simulink model "CASMain"  (R2023b)
settings: Solver=FixedStepAuto  StartTime=0.0  StopTime=10.0  FixedStep=0.01  RelTol=1e-3
values from neighbouring files (symbols this model uses):
  aircraft_mass = 5    [ACConfig.m]
  center_of_gravity = [0 0 0]    [ACConfig.m]
  center_of_pressure = [0 0 0]    [ACConfig.m]
  max_aileron_deflection = 30    [ACConfig.m]
  max_elevator_deflection = 30    [ACConfig.m]
  max_rudder_deflection = 30    [ACConfig.m]
  max_throttle = 100.0    (= 100)    [ACConfig.m]
  plane_latitude = 45    [ACConfig.m]
  plane_longitude = 45    [ACConfig.m]
undefined symbols (not defined in the file or in its folder): magnitude
libraries: aerolibasang x2, sim3dcameralib x2, shared6dof x1, aerolibatmos2 x1, dspmathops x1, sim3dphyssensorlib x1, sim3dlib x1, uavsim3dlib x1
settings Model: Creator=burak  LastModifiedBy=burak

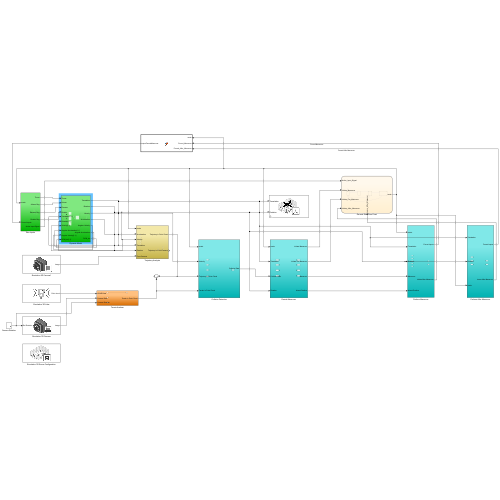
[thumbnail: Simulink's stored preview of the top-level diagram]
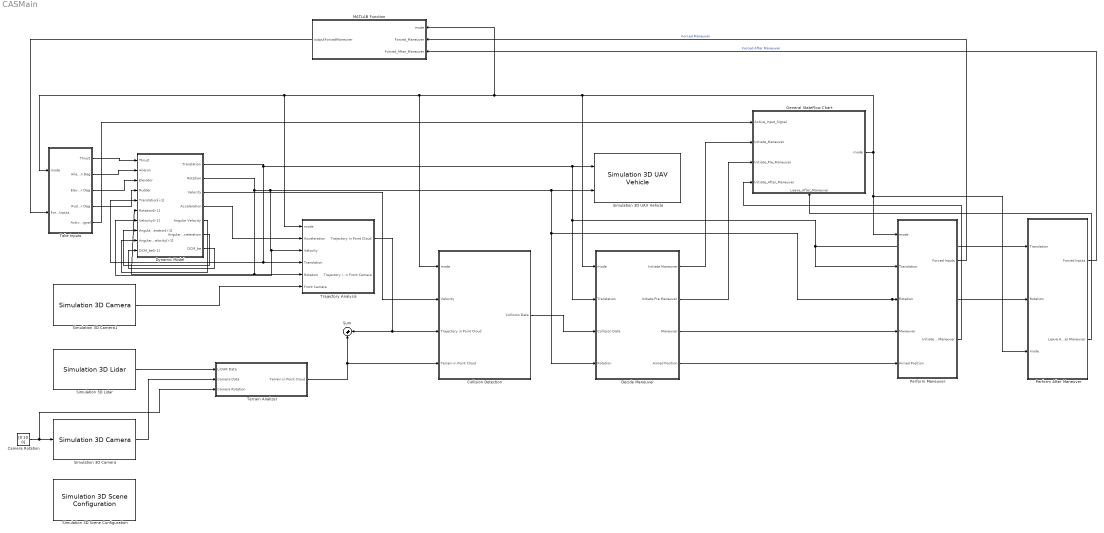
== system CASMain ==
  Camera Rotation : Constant  Value=[0 10 0]  VectorParams1D=off
  Collision Detection : Subsystem
  Decide Maneuver : Subsystem
  Dynamic Model : Subsystem
  General StateFlow Chart : Stateflow chart  TreatAsAtomicUnit=on
      settings: PortSchema="{\"entries\":[{\"content\":{\"sides\":[{\"content\":{\"connectorIds\":[\"In2\",\"In3\",\"In4\",\"In5\"]},\"type\":\"ConnectorPlacement.EquallySpacedRectSide\",\"uuid\":\"7a30dc9d-b2d0-4cd8-a09a-60d22ea8c87b\"},{\"content\":{\"connectorIds\":[\"Out1\"],\"side\":\"RIGHT\"},\"type\":\"ConnectorPlacement.EquallySpacedRectSide\",\"uuid\":\"c8b32d95-5109-4e90-83c3-dc864e15907c\"},{\"content\":{\"side\":\"TOP\"},\"type\":\"ConnectorPlacement.EquallySpacedRectSide\",\"uuid\":\"64dca0b5-bb3e-47b4-89ff-52a03a0aa1bb\"},{\"content\":{\"connectorIds\":[\"In1\"],\"side\":\"BOTTOM\"},\"type\":\"ConnectorPlacement.EquallySpacedRectSide\",\"uuid\":\"7da6c250-bc37-4c80-bd57-b46834ef644c\"}]},\"type\":\"ConnectorPlacement.EquallySpacedConnector\",\"uuid\":\"e70caf03-2dfd-4035-8f54-0e4c7b515600\"}],\"packageUris\":[\"http://schema.mathworks.com/mf0/Connector/R2020b\"],\"version\":\"1.0\"}"
  MATLAB Function : MATLAB Function  TreatAsAtomicUnit=on
  Perform After Maneuver : Subsystem
  Perform Maneuver : Subsystem
  Simulation 3D Camera : sim3dcameralib/Simulation 3D Camera  Priority=1  sensorTag=Sim3dSensor1  sensorId=1  sensorName=Sim3dSensor1  vehTagList={'Scene Origin';'SimulinkVehicle1'}  vehTag=SimulinkVehicle1  mountLoc=Origin  offsetFlag=on  tmountOffset=[0, -5, 0]  extTmount=off  rmountOffset=[0, 0, 0]  extRmount=on  FocalLength=[1109, 1109]  OpticalCenter=[640, 360]  ImageSize=[720, 1280]  RadialDistortion=[0, 0]  TangentialDistortion=[0, 0]  SensorSkew=0  DepthOutportEnabled=off  SemanticOutportEnabled=off  TransformOutportEnabled=off  SampleTime=-1  mountPoint=[0 5 0]  mountOrientation=[0 0 0]  aMode=4  ID=1
      settings: LibrarySourceBlock=uavsim3dlib/Simulation 3D Camera
  Simulation 3D Camera1 : sim3dcameralib/Simulation 3D Camera  Priority=1  sensorTag=Sim3dSensor3  sensorId=3  sensorName=Sim3dSensor3  vehTagList={'Scene Origin';'SimulinkVehicle1'}  vehTag=SimulinkVehicle1  mountLoc=Origin  offsetFlag=on  tmountOffset=[4, 0, 0]  extTmount=off  rmountOffset=[0, 0, 0]  extRmount=off  FocalLength=[1109, 1109]  OpticalCenter=[640, 360]  ImageSize=[720, 1280]  RadialDistortion=[0, 0]  TangentialDistortion=[0, 0]  SensorSkew=0  DepthOutportEnabled=off  SemanticOutportEnabled=off  TransformOutportEnabled=off  SampleTime=-1  mountPoint=[4 0 0]  mountOrientation=[0 0 0]  aMode=4  ID=3
      settings: LibrarySourceBlock=uavsim3dlib/Simulation 3D Camera
  Simulation 3D Lidar : sim3dphyssensorlib/Simulation 3D Lidar  Priority=1  sensorTag=Sim3dSensor2  sensorId=2  sensorName=Sim3dSensor2  vehTagList={'Scene Origin';'SimulinkVehicle1'}  vehTag=SimulinkVehicle1  mountLoc=Origin  offsetFlag=on  tmountOffset=[0, 0, 0]  rmountOffset=[0, 0, 0]  DetectionRange=120  RangeResolution=0.002  VerticalFOV=40  VerticalResolution=1.25  HorizontalFOV=360  HorizontalResolution=0.16  DistanceOutportEnabled=off  ReflectivityOutportEnabled=off  SemanticOutportEnabled=off  TransformOutportEnabled=off  SampleTime=-1  mountPoint=[0 0 0]  mountOrientation=[0 0 0]  aMode=4  ID=2
      settings: LibrarySourceBlock=uavsim3dlib/Simulation 3D Lidar
  Simulation 3D Scene Configuration : sim3dlib/Simulation 3D Scene Configuration  Priority=0  ProjectFormat=Default Scenes  SceneDesc=US city block  ProjectName=C:\Program Files\MATLAB\R2023b\toolbox\shared\sim3d_projects\automotive_project_windows\UE\WindowsNoEditor\VehicleSimulation.exe  ScenePath=/Game/Maps/USCityBlock  EnableOpenDRIVE=off  vehTagList={'Custom';'Scene Origin';'SimulinkVehicle1'}  vehTag=SimulinkVehicle1  FreeCameraInitialTranslation=[0, 0, 0]  FreeCameraDefaultInitialTranslation=[-6, 0, 2]  FreeCameraInitialRotation=[0, 0, 0]  FreeCameraDefaultInitialRotation=[0, -15, 0]  OpVisEn=off  Ts=0.01  EnableWindow=on  EnableRemoteAccess=off  EnableWeather=off  SunAltitude=40.0  SunAzimuth=90  clouds=10  wind=1  fog=0  rain=0  EnableGeospatial=off  OriginHeight=200  OriginLatitude=40.744652  OriginLongitude=-73.988864  MapStyle=Aerial  AdditionalAssetIDs=[]  UseAdvancedSunSky=off  SolarTime=11  TimeZone=-5  Day=21  Month=9  Year=2022  UseDaylightSavingTime=on  DSTStartDay=10  DSTStartMonth=3  DSTEndDay=3  DSTEndMonth=11  DSTSwitchHour=2  sensorTag=MainCamera1  sensorId=1  sensorName=MainCamera1  mountLoc=Origin  offsetFlag=off  tmountOffset=[0, 0, 0]  rmountOffset=[0, 0, 0]  HorizontalResolution=1280  VerticalResolution=720  HorizontalFOV=60  mountPoint=[0 0 0]  mountOrientation=[0 0 0]  aMode=4  ID=1  GeoTrigger=Inactive
      settings: LibrarySourceBlock=uavsim3dlib/Simulation 3D Scene Configuration
  Simulation 3D UAV Vehicle : uavsim3dlib/Simulation 3D UAV Vehicle  Priority=-1  Mesh=Fixed wing  MeshPath=/MathWorksUAVContent/UAVs/HexaRotorUAV/HexaRotor.HexaRotor  Color=Black  ActorName=SimulinkVehicle1  UseGlobalFrame=off  InitialTranslation=[0 0 0]  InitialRotation=[0 0 0]  InitialTranslationGlobal=[0 0 0]  InitialGeoOrigin=[0 0 0]  InitialRotationGlobal=[0 0 0]  SampleTime=-1  ActorType=SimulinkVehicle  ID=1  aMode=4  ActorTag=SimulinkVehicle1
  Sum : Sum  Inputs=|++
  Take Inputs : Subsystem
  Terrain Analizer : Subsystem
  Trajectory Analysis : Subsystem
  wires:
  Terrain Analizer/1(Terrain in Point Cloud) -> Sum/2, Collision Detection/4(Terrain in Point Cloud)
  Take Inputs/1(Thrust) -> Dynamic Model/1("Thrust ")
  Take Inputs/2(Aileron Deg) -> Dynamic Model/2(Aileron)
  Take Inputs/3(Elevator Deg) -> Dynamic Model/3(Elevator)
  Take Inputs/4(Rudder Deg) -> Dynamic Model/4(Rudder)
  Trajectory Analysis/1(Trajectory in Point Cloud) -> Sum/1, Collision Detection/3(Trajectory in Point Cloud)
  Simulation 3D Lidar/1 -> Terrain Analizer/1(LiDAR Data)
  Dynamic Model/2(Rotation) -> Dynamic Model/7(Velocity[i-1]), Trajectory Analysis/3(Velocity), Decide Maneuver/4(Rotation), Perform Maneuver/3(Rotation), Perform After Maneuver/2(Rotation), Simulation 3D UAV Vehicle/2, Trajectory Analysis/5(Rotation), Dynamic Model/6(Rotation[i-1])
  Dynamic Model/3(Velocity) -> Collision Detection/2(Velocity)
  Dynamic Model/4(Acceleration) -> Trajectory Analysis/2(Acceleration)
  Simulation 3D Camera/1 -> Terrain Analizer/2(Camera Data)
  Camera Rotation/1 -> Terrain Analizer/3(Camera Rotation), Simulation 3D Camera/1
  Dynamic Model/1(Translation) -> Decide Maneuver/2(Translation), Perform Maneuver/2(Translation), Perform After Maneuver/1(Translation), Simulation 3D UAV Vehicle/1, Trajectory Analysis/4(Translation), Dynamic Model/5(Translation[i-1])
  Simulation 3D Camera1/1 -> Trajectory Analysis/6(Front Camera)
  Collision Detection/1(Collision Data) -> Decide Maneuver/3(Collision Data)
  Decide Maneuver/1(Initiate Maneuver) -> General StateFlow Chart/3(Initiate_Maneuver)
  Take Inputs/5(Active Input Signal) -> General StateFlow Chart/2(Active_Input_Signal)
  General StateFlow Chart/1(mode) -> Perform After Maneuver/3(mode), Perform Maneuver/1(mode), Collision Detection/1(mode), Trajectory Analysis/1(mode), Take Inputs/1(mode), MATLAB Function/1(mode), Decide Maneuver/1(mode)
  Decide Maneuver/3(Maneuver) -> Perform Maneuver/4(Maneuver)
  Decide Maneuver/4(Aimed Position) -> Perform Maneuver/5(Aimed Position)
  Decide Maneuver/2(Initiate Pre Maneuver) -> General StateFlow Chart/4(Initiate_Pre_Maneuver)
  Perform Maneuver/1(Forced Inputs) -> MATLAB Function/2(Forced_Maneuver)  "Forced Maneuver"
  Perform Maneuver/2(Initiate After Maneuver) -> General StateFlow Chart/5(Initiate_After_Maneuver)
  Perform After Maneuver/1(Forced Inputs) -> MATLAB Function/3(Forced_After_Maneuver)  "Forced After Maneuver"
  MATLAB Function/1(outputForcedManeuver) -> Take Inputs/2(Forced Inputs)
  Perform After Maneuver/2(Leave After Maneuver) -> General StateFlow Chart/1(Leave_After_Maneuver)
  Dynamic Model/5(Angular Velocity) -> Dynamic Model/9(Angular Velocity[i-1])
  Dynamic Model/6(Angular Acceleration) -> Dynamic Model/8(Angular Acceleration[i-1])
  Dynamic Model/7(DCM_be) -> Dynamic Model/10(DCM_be[i-1])

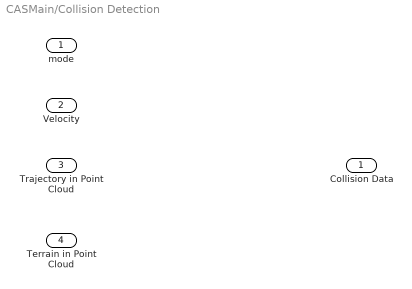
== system CASMain/Collision Detection ==
  mode : Inport
  Velocity : Inport  Port=2
  Trajectory in Point Cloud : Inport  Port=3
  Terrain in Point Cloud : Inport  Port=4
  Collision Data : Outport

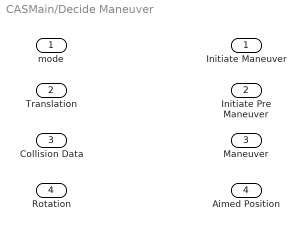
== system CASMain/Decide Maneuver ==
  mode : Inport
  Translation : Inport  Port=2
  Collision Data : Inport  Port=3
  Rotation : Inport  Port=4
  Initiate Maneuver : Outport
  Initiate Pre Maneuver : Outport  Port=2
  Maneuver : Outport  Port=3
  Aimed Position : Outport  Port=4

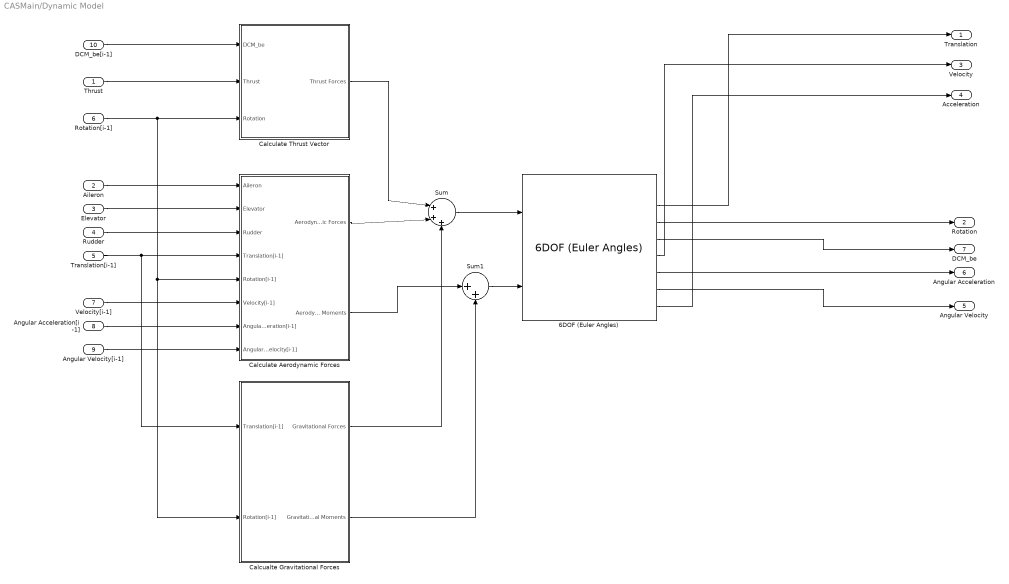
== system CASMain/Dynamic Model ==
  "Thrust " : Inport
  Aileron : Inport  Port=2
  Elevator : Inport  Port=3
  Rudder : Inport  Port=4
  Translation[i-1] : Inport  Port=5
  Rotation[i-1] : Inport  Port=6
  Velocity[i-1] : Inport  Port=7
  Angular Acceleration[i-1] : Inport  Port=8
  Angular Velocity[i-1] : Inport  Port=9
  DCM_be[i-1] : Inport  Port=10
  6DOF (Euler Angles) : shared6dof/6DOF (Euler Angles)  units=Metric (MKS)  mtype=Fixed  rep=Euler Angles  xme_0=[0 0 0.275]  Vm_0=[0 0 0]  eul_0=[0 0 0]  pm_0=[0 0 0]  mass_0=aircraft_mass  mass_e=0.5  mass_f=2.0  inertia=eye(3)  inertia_e=eye(3)  inertia_f=2*eye(3)  k_quat=1.0  vre_flag=on  abi_flag=off  aMode=0  xme_statename=''  Vm_statename=''  eul_statename=''  quat_statename=''  pm_statename=''  mass_statename=''
  Calcualte Gravitational Forces : Subsystem
  Calculate Aerodynamic Forces : Subsystem
  Calculate Thrust Vector : Subsystem
  Sum : Sum  Inputs=|+++
  Sum1 : Sum  Inputs=|++
  Translation : Outport
  Rotation : Outport  Port=2
  Velocity : Outport  Port=3
  Acceleration : Outport  Port=4
  Angular Velocity : Outport  Port=5
  Angular Acceleration : Outport  Port=6
  DCM_be : Outport  Port=7
  wires:
  6DOF (Euler Angles)/2 -> Translation/1
  6DOF (Euler Angles)/8 -> Acceleration/1
  "Thrust "/1 -> Calculate Thrust Vector/2(Thrust)
  Rotation[i-1]/1 -> Calcualte Gravitational Forces/2(Rotation[i-1]), Calculate Aerodynamic Forces/5(Rotation[i-1]), Calculate Thrust Vector/3(Rotation)
  6DOF (Euler Angles)/3 -> Rotation/1
  Aileron/1 -> Calculate Aerodynamic Forces/1(Aileron)
  Elevator/1 -> Calculate Aerodynamic Forces/2(Elevator)
  Rudder/1 -> Calculate Aerodynamic Forces/3(Rudder)
  Translation[i-1]/1 -> Calculate Aerodynamic Forces/4(Translation[i-1]), Calcualte Gravitational Forces/1(Translation[i-1])
  Velocity[i-1]/1 -> Calculate Aerodynamic Forces/6(Velocity[i-1])
  6DOF (Euler Angles)/6 -> Angular Acceleration/1
  6DOF (Euler Angles)/7 -> Angular Velocity/1
  Angular Acceleration[i-1]/1 -> Calculate Aerodynamic Forces/7(Angular Acceleration[i-1])
  Angular Velocity[i-1]/1 -> Calculate Aerodynamic Forces/8(Angular Velocity[i-1])
  Sum/1 -> 6DOF (Euler Angles)/1
  Calculate Thrust Vector/1(Thrust Forces) -> Sum/1
  Calcualte Gravitational Forces/1(Gravitational Forces) -> Sum/3
  Calcualte Gravitational Forces/2(Gravitational Moments) -> Sum1/2
  Sum1/1 -> 6DOF (Euler Angles)/2
  Calculate Aerodynamic Forces/1(Aerodynamic Forces) -> Sum/2
  Calculate Aerodynamic Forces/2(Aerodynamic Moments) -> Sum1/1
  6DOF (Euler Angles)/5 -> Velocity/1
  6DOF (Euler Angles)/4 -> DCM_be/1
  DCM_be[i-1]/1 -> Calculate Thrust Vector/1(DCM_be)

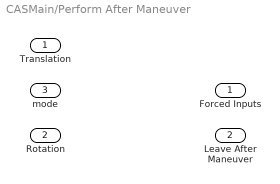
== system CASMain/Perform After Maneuver ==
  Translation : Inport
  Rotation : Inport  Port=2
  mode : Inport  Port=3
  Forced Inputs : Outport
  Leave After Maneuver : Outport  Port=2

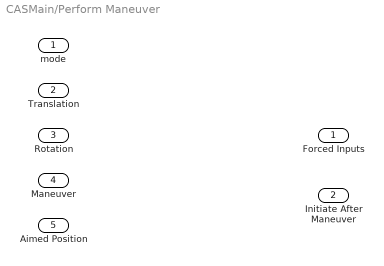
== system CASMain/Perform Maneuver ==
  mode : Inport
  Translation : Inport  Port=2
  Rotation : Inport  Port=3
  Maneuver : Inport  Port=4
  Aimed Position : Inport  Port=5
  Forced Inputs : Outport
  Initiate After Maneuver : Outport  Port=2

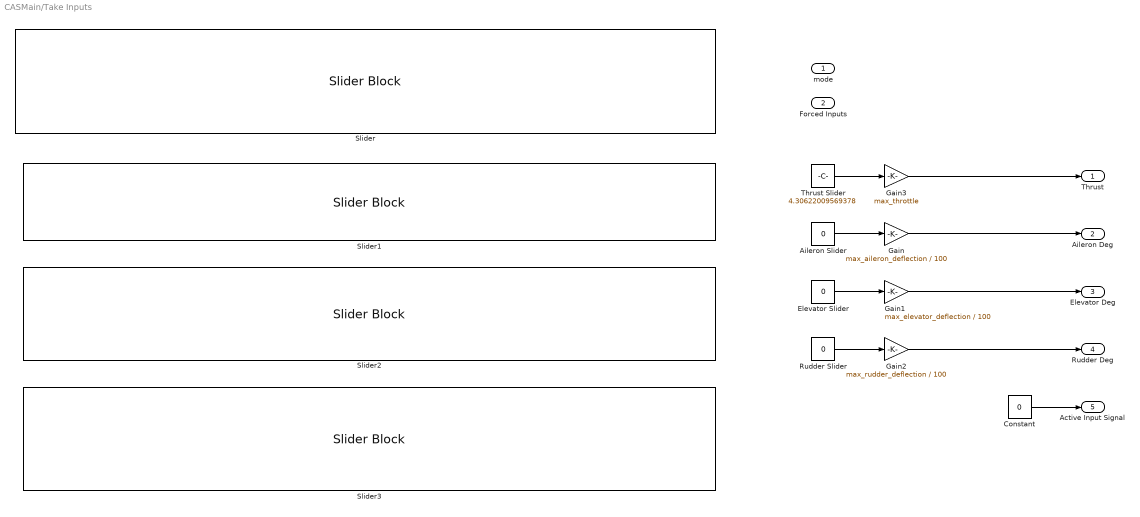
== system CASMain/Take Inputs ==
  mode : Inport
  Forced Inputs : Inport  Port=2
  Aileron Slider : Constant  Value=0
  Constant : Constant  Value=0  OutDataTypeStr=boolean
  Elevator Slider : Constant  Value=0
  Gain : Gain  Gain=max_aileron_deflection / 100
  Gain1 : Gain  Gain=max_elevator_deflection / 100
  Gain2 : Gain  Gain=max_rudder_deflection / 100
  Gain3 : Gain  Gain=max_throttle
  Rudder Slider : Constant  Value=0
  Slider : SliderBlock
  Slider1 : SliderBlock  ScaleMin=-100
  Slider2 : SliderBlock  ScaleMin=-100
  Slider3 : SliderBlock  ScaleMin=-100
  Thrust Slider : Constant  Value=4.30622009569378
  Thrust : Outport
  Aileron Deg : Outport  Port=2
  Elevator Deg : Outport  Port=3
  Rudder Deg : Outport  Port=4
  Active Input Signal : Outport  Port=5
  wires:
  Aileron Slider/1 -> Gain/1
  Gain/1 -> Aileron Deg/1
  Elevator Slider/1 -> Gain1/1
  Rudder Slider/1 -> Gain2/1
  Gain1/1 -> Elevator Deg/1
  Gain2/1 -> Rudder Deg/1
  Thrust Slider/1 -> Gain3/1
  Gain3/1 -> Thrust/1
  Constant/1 -> Active Input Signal/1

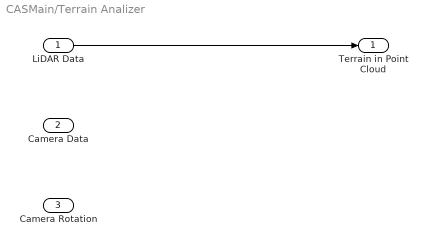
== system CASMain/Terrain Analizer ==
  LiDAR Data : Inport
  Camera Data : Inport  Port=2
  Camera Rotation : Inport  Port=3
  Terrain in Point Cloud : Outport
  wires:
  LiDAR Data/1 -> Terrain in Point Cloud/1

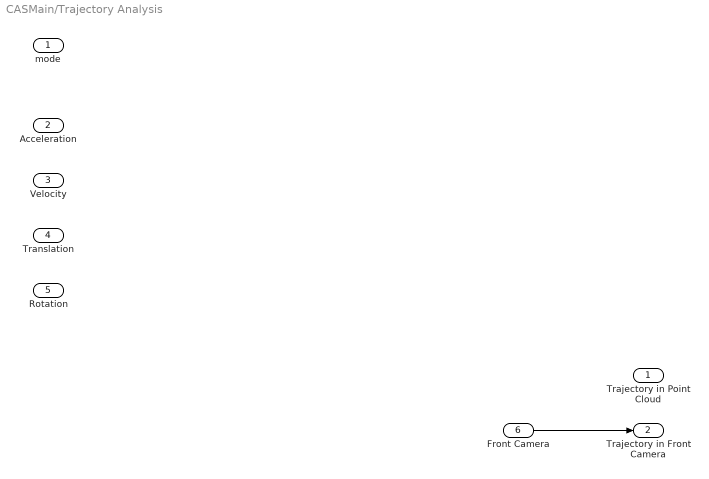
== system CASMain/Trajectory Analysis ==
  mode : Inport
  Acceleration : Inport  Port=2
  Velocity : Inport  Port=3
  Translation : Inport  Port=4
  Rotation : Inport  Port=5
  Front Camera : Inport  Port=6
  Trajectory in Point Cloud : Outport
  Trajectory in Front Camera : Outport  Port=2
  wires:
  Front Camera/1 -> Trajectory in Front Camera/1

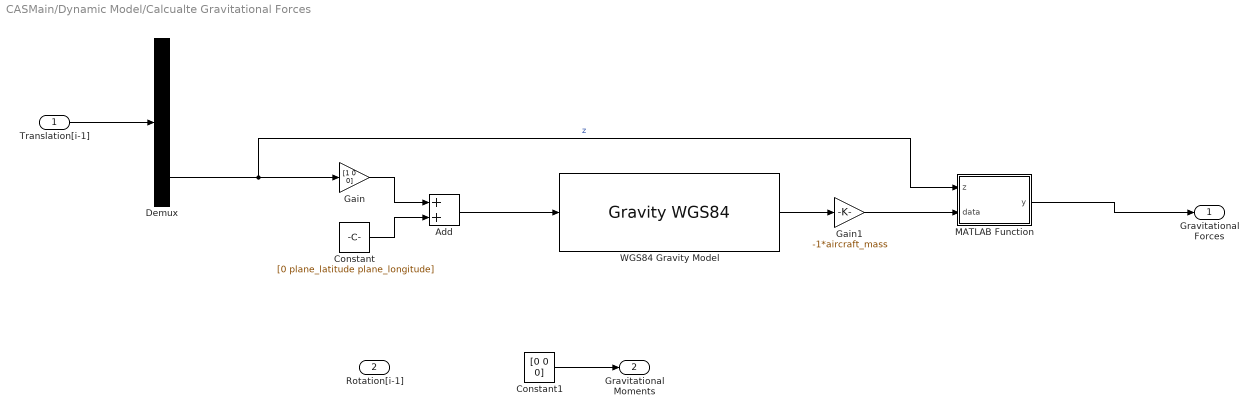
== system CASMain/Dynamic Model/Calcualte Gravitational Forces ==
  Translation[i-1] : Inport
  Rotation[i-1] : Inport  Port=2
  Add : Sum
  Constant : Constant  Value=[0 plane_latitude plane_longitude]  VectorParams1D=off
  Constant1 : Constant  Value=[0 0 0]
  Demux : Demux  Outputs=3
  Gain : Gain  Gain=[1 0 0]
  Gain1 : Gain  Gain=-1*aircraft_mass
  MATLAB Function : MATLAB Function  TreatAsAtomicUnit=on
  "WGS84 Gravity Model  " : GravityWGS84
  Gravitational Forces : Outport
  Gravitational Moments : Outport  Port=2
  wires:
  Translation[i-1]/1 -> Demux/1
  Gain/1 -> Add/1
  Constant/1 -> Add/2
  Add/1 -> "WGS84 Gravity Model  "/1
  "WGS84 Gravity Model  "/1 -> Gain1/1
  Demux/3 -> MATLAB Function/1(z), Gain/1  "z"
  Gain1/1 -> MATLAB Function/2(data)
  MATLAB Function/1(y) -> Gravitational Forces/1
  Constant1/1 -> Gravitational Moments/1

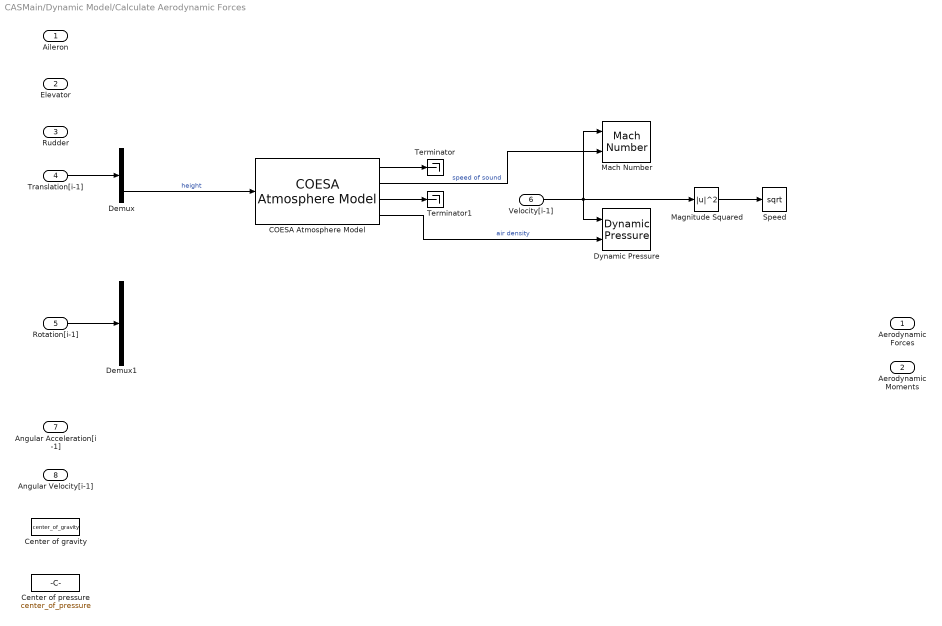
== system CASMain/Dynamic Model/Calculate Aerodynamic Forces ==
  Aileron : Inport
  Elevator : Inport  Port=2
  Rudder : Inport  Port=3
  Translation[i-1] : Inport  Port=4
  Rotation[i-1] : Inport  Port=5
  Velocity[i-1] : Inport  Port=6
  Angular Acceleration[i-1] : Inport  Port=7
  Angular Velocity[i-1] : Inport  Port=8
  COESA Atmosphere Model : aerolibatmos2/COESA Atmosphere Model  units=Metric (MKS)  spec=1976 COESA-extended U.S. Standard Atmosphere  model=Profile  profile_var=High temperature  profile_percent=1%  profile_alt=5 km (16404 ft)  envelope_var=High temperature  envelope_percent=1%  action=Warning
  Center of gravity : Constant  Value=center_of_gravity
  Center of pressure : Constant  Value=center_of_pressure
  Demux : Demux  Outputs=3
  Demux1 : Demux  Outputs=3
  Dynamic Pressure : aerolibasang/Dynamic Pressure
  Mach Number : aerolibasang/Mach Number
  Magnitude Squared : Math  Operator=magnitude^2
  Speed : Sqrt
  Terminator : Terminator
  Terminator1 : Terminator
  Aerodynamic Forces : Outport
  Aerodynamic Moments : Outport  Port=2
  wires:
  Velocity[i-1]/1 -> Magnitude Squared/1, Mach Number/1, Dynamic Pressure/1
  Translation[i-1]/1 -> Demux/1
  Demux/3 -> COESA Atmosphere Model/1  "height"
  COESA Atmosphere Model/2 -> Mach Number/2  "speed of sound"
  COESA Atmosphere Model/4 -> Dynamic Pressure/2  "air density"
  Rotation[i-1]/1 -> Demux1/1
  Magnitude Squared/1 -> Speed/1
  COESA Atmosphere Model/1 -> Terminator/1
  COESA Atmosphere Model/3 -> Terminator1/1

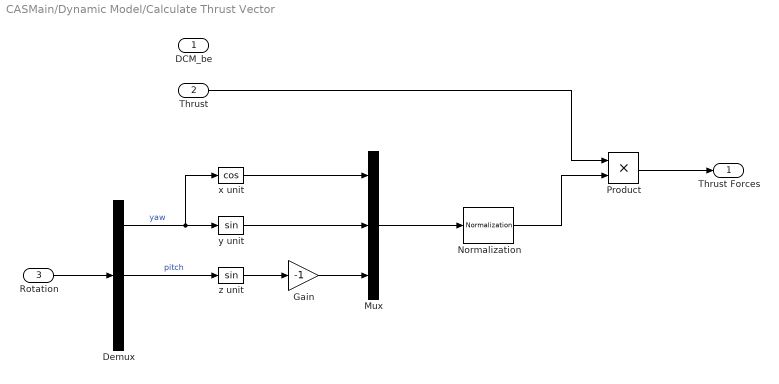
== system CASMain/Dynamic Model/Calculate Thrust Vector ==
  DCM_be : Inport
  Thrust : Inport  Port=2
  Rotation : Inport  Port=3
  Demux : Demux  Outputs=3
  Gain : Gain  Gain=-1
  Mux : Mux  Inputs=3
  Normalization : dspmathops/Normalization  NormType=Squared 2-norm  Bias=1e-10  NormOver=Each column  Dimension=1  roundingMode=Floor  overflowMode=off  accumDataTypeStr=Inherit: Same as product output  accumLastDataTypeStr=Inherit: Same as product output  outputDataTypeStr=Inherit: Same as product output  outputMin=[]  outputMax=[]  outputLastDataTypeStr=Inherit: Same as product output
  Product : Product
  x unit : Trigonometry  Operator=cos
  y unit : Trigonometry
  z unit : Trigonometry
  Thrust Forces : Outport
  wires:
  Thrust/1 -> Product/1
  Rotation/1 -> Demux/1
  Demux/2 -> z unit/1  "pitch"
  Demux/1 -> x unit/1, y unit/1  "yaw"
  Product/1 -> Thrust Forces/1
  x unit/1 -> Mux/1
  y unit/1 -> Mux/2
  z unit/1 -> Gain/1
  Gain/1 -> Mux/3
  Mux/1 -> Normalization/1
  Normalization/1 -> Product/2

== matlab function CASMain/Dynamic Model/Calcualte Gravitational Forces/MATLAB Function ==
  data: z input; y output; data input
function y = fcn(z, data)

if z <= 0.275
    y = [0 0 0];
else
    y = data;
end

== matlab function CASMain/MATLAB Function ==
  data: mode input; outputForcedManeuver output; Forced_Maneuver input; Forced_After_Maneuver input
function outputForcedManeuver = fnc(mode, Forced_Maneuver, Forced_After_Maneuver)

if mode == 2
    outputForcedManeuver = Forced_Maneuver;
elseif mode == 3
    outputForcedManeuver = Forced_After_Maneuver;
else
    outputForcedManeuver = -1;
end

== stateflow chart CASMain/General StateFlow Chart ==
  state ManualInput
    entry:
    mode = 0;
  state PreManeuver
    entry:
    mode = 1;
  state Maneuver
    entry:
    mode = 2;
  state AfterManeuver
    entry:
    mode = 3;
  (default) -> ManualInput : {mode=0;}
  ManualInput -> PreManeuver : [Initiate_Pre_Maneuver == 1]
  PreManeuver -> Maneuver [order 2] : [Initiate_Maneuver == 1]
  Maneuver -> AfterManeuver [order 2] : [Initiate_After_Maneuver == 1]
  PreManeuver -> ManualInput [order 1] : [Active_Input_Signal == 1]
  AfterManeuver -> ManualInput : [Active_Input_Signal == 1 | Leave_After_Maneuver == 1]
  Maneuver -> ManualInput [order 1] : [Active_Input_Signal == 1]
  data: Leave_After_Maneuver input; Active_Input_Signal input; Initiate_Maneuver input; mode output; Initiate_Pre_Maneuver input; Initiate_After_Maneuver input
